simulink model "sedemo_ipswitch_v_pathcombiner"  (Simulink 7.5)
settings: Solver=VariableStepDiscrete  StartTime=0.0  StopTime=10.0  MaxStep=inf  RelTol=1e-3
undefined symbols (not defined in the file or in its folder): slcm
libraries: simeventsgenerators1 x6, simeventsattributes2 x6, simeventssink1 x4, simeventsrouting1 x2
settings Model: Creator=The MathWorks Inc.  ExtModeAutoUpdateStatusClock=off
settings DataIOCC: SaveOutput=off  SaveTime=off
settings OptimizationCC: InitFltsAndDblsToZero=on
settings DebuggingCC: AlgebraicLoopMsg=error  SaveWithParameterizedLinksMsg=none  SignalResolutionControl=TryResolveAllWithWarning  SolverPrmCheckMsg=none  MultiTaskDSMMsg=warning  MultiTaskCondExecSysMsg=none  SigSpecEnsureSampleTimeMsg=none  StrictBusMsg=None
settings RTWCC: IncludeERTFirstTime=on
settings GRTTargetCC: TargetFcnLib=ansi_tfl_tmw.mat
settings SimEventsCC: propIdentEventSeed=12345678  propDiagAttribOutput=1  propDiagFcnCallOutput=1  propDiagStatOutput=0

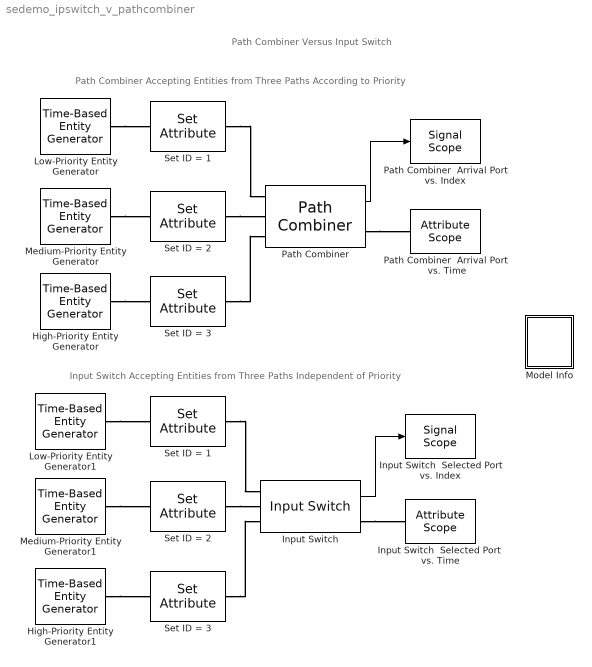
== system sedemo_ipswitch_v_pathcombiner ==
  note: Path Combiner Accepting Entities from Three Paths According to Priority
  note: Input Switch Accepting Entities from Three Paths Independent of Priority
  note: Path Combiner Versus Input Switch
  High-Priority Entity Generator : simeventsgenerators1/Entity Generators/Time-Based Entity Generator  Priority=1  DialogController=des_ddg_create  DialogControllerArgs=DataTag1  SystemSampleTime=-1  GenerateEntitiesUpon=Intergeneration time from dialog  Distribution=Constant  Minimum=0  Maximum=1  Mean=1  InitialSeed=12345  Period=1  PriorityEntityGeneration=1  GenerateEntityAtSimulationStart=on  ResponseWhenBlocked=Pause generation  ResponseWhenUnblocked=Immediate restart  EntityType=Standard  StatNumberDeparted=Off  StatPendingEntity=Off  StatAverageIntergenerationTime=Off
  High-Priority Entity Generator1 : simeventsgenerators1/Entity Generators/Time-Based Entity Generator  Priority=1  DialogController=des_ddg_create  DialogControllerArgs=DataTag3  SystemSampleTime=-1  GenerateEntitiesUpon=Intergeneration time from dialog  Distribution=Constant  Minimum=0  Maximum=1  Mean=1  InitialSeed=12345  Period=1  PriorityEntityGeneration=1  GenerateEntityAtSimulationStart=on  ResponseWhenBlocked=Pause generation  ResponseWhenUnblocked=Immediate restart  EntityType=Standard  StatNumberDeparted=Off  StatPendingEntity=Off  StatAverageIntergenerationTime=Off
  Input Switch : simeventsrouting1/Input Switch  Priority=1  SystemSampleTime=-1  NumberInputPorts=3  SwitchingCriterion=Round robin  InitialSeed=23456  SpecifyEventPriority=off  PriorityInputSwitchSelectPort=4000  StatNumberDeparted=Off  StatLastArrivalPort=On  EvaluatedNumPorts=3
      settings: AttributesFormatString=Policy: %<SwitchingCriterion>
  Input Switch  Selected Port  vs. Time : simeventssink1/Attribute Scope  Priority=1  SystemSampleTime=-1  PlotType=Continuous  InputType=Attribute  NumInputs=1  AttributeNameY=ID  XInputOptionSignal=Event time  XInputOptionEntity=Event time  AttributeNameX=Count  EnableEntityOutport=off  XMin=0  XMax=10  XLimitExceededOption=Stretch axis limits  YLimitExceededOption=Stretch axis limits  AxisGrid=on  AxisLegend=off  LineDisables=""  LineColors=b  LineStyles=-  LineMarkers=o  OpenScopeAtSimStart=on  Title=Input Switch Selected Port vs. Time  YLabel=Selected Port  XLabel=Time  FigurePosition=[643 35 376 111]  AxisZoom=off  DataStoreOption=Limited  DataPointsLimit=10000  StatNumberArrived=Off  ShowCountPlotted=off  ShowToolbar=on
      settings: YMin=1  YMax=3
  Input Switch  Selected Port vs. Index : simeventssink1/Signal Scope  Priority=1  SystemSampleTime=-1  PlotType=Stair  InputType=Signal  NumInputs=1  AttributeNameY=Count  XInputOptionSignal=Index  XInputOptionEntity=Event time  AttributeNameX=Count  EnableEntityOutport=on  XMin=0  XMax=10  XLimitExceededOption=Stretch axis limits  YLimitExceededOption=Stretch axis limits  AxisGrid=on  AxisLegend=off  LineDisables=""  LineColors=b  LineStyles=-  LineMarkers=.  OpenScopeAtSimStart=on  Title=Input Switch Selected Port vs. Index  YLabel=Selected Port  XLabel=Index  FigurePosition=[643 215 376 113]  AxisZoom=off  DataStoreOption=Limited  DataPointsLimit=10000  StatNumberArrived=Off  ShowCountPlotted=off  ShowToolbar=on
      settings: YMin=1  YMax=3
  Low-Priority Entity Generator : simeventsgenerators1/Entity Generators/Time-Based Entity Generator  Priority=1  DialogController=des_ddg_create  DialogControllerArgs=DataTag8  SystemSampleTime=-1  GenerateEntitiesUpon=Intergeneration time from dialog  Distribution=Constant  Minimum=0  Maximum=1  Mean=1  InitialSeed=12345  Period=1  PriorityEntityGeneration=3  GenerateEntityAtSimulationStart=on  ResponseWhenBlocked=Pause generation  ResponseWhenUnblocked=Immediate restart  EntityType=Standard  StatNumberDeparted=Off  StatPendingEntity=Off  StatAverageIntergenerationTime=Off
  Low-Priority Entity Generator1 : simeventsgenerators1/Entity Generators/Time-Based Entity Generator  Priority=1  DialogController=des_ddg_create  DialogControllerArgs=DataTag10  SystemSampleTime=-1  GenerateEntitiesUpon=Intergeneration time from dialog  Distribution=Constant  Minimum=0  Maximum=1  Mean=1  InitialSeed=12345  Period=1  PriorityEntityGeneration=3  GenerateEntityAtSimulationStart=on  ResponseWhenBlocked=Pause generation  ResponseWhenUnblocked=Immediate restart  EntityType=Standard  StatNumberDeparted=Off  StatPendingEntity=Off  StatAverageIntergenerationTime=Off
  Medium-Priority Entity Generator : simeventsgenerators1/Entity Generators/Time-Based Entity Generator  Priority=1  DialogController=des_ddg_create  DialogControllerArgs=DataTag12  SystemSampleTime=-1  GenerateEntitiesUpon=Intergeneration time from dialog  Distribution=Constant  Minimum=0  Maximum=1  Mean=1  InitialSeed=12345  Period=1  PriorityEntityGeneration=2  GenerateEntityAtSimulationStart=on  ResponseWhenBlocked=Pause generation  ResponseWhenUnblocked=Immediate restart  EntityType=Standard  StatNumberDeparted=Off  StatPendingEntity=Off  StatAverageIntergenerationTime=Off
  Medium-Priority Entity Generator1 : simeventsgenerators1/Entity Generators/Time-Based Entity Generator  Priority=1  DialogController=des_ddg_create  DialogControllerArgs=DataTag14  SystemSampleTime=-1  GenerateEntitiesUpon=Intergeneration time from dialog  Distribution=Constant  Minimum=0  Maximum=1  Mean=1  InitialSeed=12345  Period=1  PriorityEntityGeneration=2  GenerateEntityAtSimulationStart=on  ResponseWhenBlocked=Pause generation  ResponseWhenUnblocked=Immediate restart  EntityType=Standard  StatNumberDeparted=Off  StatPendingEntity=Off  StatAverageIntergenerationTime=Off
  Model Info : Subsystem  LoadFcn=slcm LoadBlock;  InitFcn=slcm('UpdateAllCMBlocksInThisModelInit')  mask(CMBlock){InitialSaveTempField=, InitialBlockCM=None, BlockCM=None, Frame=on, SaveTempField=, DisplayStringWithTags=Info, MaskDisplayString=Info, HorizontalTextAlignment=Center, LeftAlignmentValue=0.5, SourceBlockDiagram=sedemo_ipswitch_v_pathcombiner, TagMaxNumber=20, CMTag1=, CMTag2=, CMTag3=, CMTag4=, CMTag5=, CMTag6=, CMTag7=, CMTag8=, CMTag9=, CMTag10=, CMTag11=, CMTag12=, CMTag13=, CMTag14=, CMTag15=, CMTag16=, CMTag17=, CMTag18=, CMTag19=, CMTag20=}
      mask help: This block allows revision control information to be displayed within the model.
      settings: CopyFcn=slcm CopyBlock;  DeleteFcn=slcm Cancel;  PostSaveFcn=slcm('UpdateAllCMBlocksInThisModel')  NameChangeFcn=slcm Rename;  OpenFcn=open_system([gcb '/Information'])
      mask Display: text(str2num(LeftAlignmentValue), 0.5, MaskDisplayString, 'HorizontalAlignment', HorizontalTextAlignment)
  Path Combiner : simeventsrouting1/Path Combiner  Priority=1  SystemSampleTime=-1  NumberInputPorts=3  InputPortPrecedence=IN1 port  InitialSeed=45678  SpecifyEventPriority=off  PriorityPathCombinerPortPrecedenceSelection=4100  StatNumberDeparted=Off  StatLastArrivalPort=On  EvaluatedNumPorts=3
  Path Combiner  Arrival Port  vs. Time : simeventssink1/Attribute Scope  Priority=1  SystemSampleTime=-1  PlotType=Continuous  InputType=Attribute  NumInputs=1  AttributeNameY=ID  XInputOptionSignal=Event time  XInputOptionEntity=Event time  AttributeNameX=Count  EnableEntityOutport=off  XMin=0  XMax=10  XLimitExceededOption=Stretch axis limits  YLimitExceededOption=Stretch axis limits  AxisGrid=on  AxisLegend=off  LineDisables=""  LineColors=b  LineStyles=-  LineMarkers=o  OpenScopeAtSimStart=on  Title=Path Combiner Selected Port vs. Time  YLabel=Selected Port  XLabel=Time  FigurePosition=[643 400 376 113]  AxisZoom=off  DataStoreOption=Limited  DataPointsLimit=10000  StatNumberArrived=Off  ShowCountPlotted=off  ShowToolbar=on
      settings: YMin=1  YMax=3
  Path Combiner  Arrival Port vs. Index : simeventssink1/Signal Scope  Priority=1  SystemSampleTime=-1  PlotType=Stair  InputType=Signal  NumInputs=1  AttributeNameY=Count  XInputOptionSignal=Index  XInputOptionEntity=Event time  AttributeNameX=Count  EnableEntityOutport=on  XMin=0  XMax=10  XLimitExceededOption=Stretch axis limits  YLimitExceededOption=Stretch axis limits  AxisGrid=on  AxisLegend=off  LineDisables=""  LineColors=b  LineStyles=-  LineMarkers=.  OpenScopeAtSimStart=on  Title=Path Combiner Selected Port vs. Index  YLabel=Selected Port  XLabel=Index  FigurePosition=[643 585 376 113]  AxisZoom=off  DataStoreOption=Limited  DataPointsLimit=10000  StatNumberArrived=Off  ShowCountPlotted=off  ShowToolbar=on
      settings: YMin=1  YMax=3
  Set ID = 1 : simeventsattributes2/Set Attribute  Priority=1  DialogController=des_ddg_create  DialogControllerArgs=DataTag19  SystemSampleTime=-1  AttributeFrom=Dialog  AttributeName=ID  AttributeTreatAsVector=1  AttributeValue=1  AttributeCreate=on  StatNumberDeparted=Off  EvaluatedAttributeValue={1}
  "Set ID = 1 " : simeventsattributes2/Set Attribute  Priority=1  DialogController=des_ddg_create  DialogControllerArgs=DataTag21  SystemSampleTime=-1  AttributeFrom=Dialog  AttributeName=ID  AttributeTreatAsVector=1  AttributeValue=1  AttributeCreate=on  StatNumberDeparted=Off  EvaluatedAttributeValue={1}
  Set ID = 2 : simeventsattributes2/Set Attribute  Priority=1  DialogController=des_ddg_create  DialogControllerArgs=DataTag23  SystemSampleTime=-1  AttributeFrom=Dialog  AttributeName=ID  AttributeTreatAsVector=1  AttributeValue=2  AttributeCreate=on  StatNumberDeparted=Off  EvaluatedAttributeValue={2}
  "Set ID = 2 " : simeventsattributes2/Set Attribute  Priority=1  DialogController=des_ddg_create  DialogControllerArgs=DataTag25  SystemSampleTime=-1  AttributeFrom=Dialog  AttributeName=ID  AttributeTreatAsVector=1  AttributeValue=2  AttributeCreate=on  StatNumberDeparted=Off  EvaluatedAttributeValue={2}
  Set ID = 3 : simeventsattributes2/Set Attribute  Priority=1  DialogController=des_ddg_create  DialogControllerArgs=DataTag27  SystemSampleTime=-1  AttributeFrom=Dialog  AttributeName=ID  AttributeTreatAsVector=1  AttributeValue=3  AttributeCreate=on  StatNumberDeparted=Off  EvaluatedAttributeValue={3}
  "Set ID = 3 " : simeventsattributes2/Set Attribute  Priority=1  DialogController=des_ddg_create  DialogControllerArgs=DataTag29  SystemSampleTime=-1  AttributeFrom=Dialog  AttributeName=ID  AttributeTreatAsVector=1  AttributeValue=3  AttributeCreate=on  StatNumberDeparted=Off  EvaluatedAttributeValue={3}
  wires:
  Input Switch/1 -> Input Switch  Selected Port vs. Index/1
  Path Combiner/1 -> Path Combiner  Arrival Port vs. Index/1
  connections:
  "Set ID = 1 "/RConn1 -- Input Switch/LConn1
  "Set ID = 2 "/RConn1 -- Input Switch/LConn2
  "Set ID = 3 "/RConn1 -- Input Switch/LConn3
  Input Switch/RConn1 -- Input Switch  Selected Port  vs. Time/LConn1
  High-Priority Entity Generator/RConn1 -- Set ID = 3/LConn1
  Medium-Priority Entity Generator/RConn1 -- Set ID = 2/LConn1
  Low-Priority Entity Generator/RConn1 -- Set ID = 1/LConn1
  Set ID = 1/RConn1 -- Path Combiner/LConn1
  Set ID = 2/RConn1 -- Path Combiner/LConn2
  Set ID = 3/RConn1 -- Path Combiner/LConn3
  Path Combiner/RConn1 -- Path Combiner  Arrival Port  vs. Time/LConn1
  Low-Priority Entity Generator1/RConn1 -- "Set ID = 1 "/LConn1
  Medium-Priority Entity Generator1/RConn1 -- "Set ID = 2 "/LConn1
  High-Priority Entity Generator1/RConn1 -- "Set ID = 3 "/LConn1

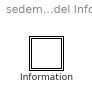
== system sedemo_ipswitch_v_pathcombiner/Model Info ==
  Information : Subsystem

== system sedemo_ipswitch_v_pathcombiner/Model Info/Information ==
  note: Path Combiner Versus Input Switch
  note: This demo contrasts the Path Combiner block and the Input Switch block. The
      | Path Combiner block accepts entities as they arrive at any port. The Input Switch
      | accepts entities only from the port that is selected, where the selection changes
      | in a round-robin fashion with the passage of each entity.
      |
      | In the upper part of the model, entities from the high-priority entity generator
      | arrive at the Path Combiner block before simultaneously generated entities having
      | a lower priority. The plots from the Path Combiner block reflect the prioritized
      | order in which the entities arrive at and pass through the Path Combiner block.
      |
      | In the lower part of the model, the Input Switch block permits arrival only at  the
      | selected port. The prioritization of entity generation events does not influence the
      | switch block. The plots from the Input Switch block reflect the ascending
      | (round-robin) order in which the entities are selected by the Input Switch block.
